simulink model "pidcontrollers"  (R2023a)
settings: Solver=FixedStepAuto  StartTime=0.0  StopTime=50  RelTol=1e-3  EnableMultiTasking=on
settings Model: Creator=dell  LastModifiedBy=mluser
settings SolverCC: AlgebraicLoopSolver=TrustRegion
settings DataIOCC: LimitDataPoints=on  SaveFormat=Array  ReturnWorkspaceOutputs=off
settings OptimizationCC: LifeSpan=inf
settings DebuggingCC: SignalInfNanChecking=error  UnconnectedInputMsg=warning  UnconnectedOutputMsg=warning  UnconnectedLineMsg=warning  SFUnexpectedBacktrackingDiag=warning  SFNoUnconditionalDefaultTransitionDiag=warning  SFExecutionAtInitializationDiag=none  ArithmeticOperatorsInVariantConditions=warning
settings HardwareCC: ProdBitPerPointer=32  ProdBitPerSizeT=32  ProdBitPerPtrDiffT=32  ProdLargestAtomicFloat=None  ProdIntDivRoundTo=Undefined  ProdEndianess=Unspecified  ProdWordSize=32  ProdHWDeviceType=32-bit Generic
settings ModelReferenceCC: PropagateSignalLabelsOutOfModel=off
settings SFSimCC: SimUseLocalCustomCode=off  CustomCodeUndefinedFunction=UseInterfaceOnly
settings RTWCC: RTWUseLocalCustomCode=off
settings CodeAppCC: StateflowObjectComments=on
settings GRTTargetCC: TargetLangStandard=C89/C90 (ANSI)
settings ConfigComp: CovMetricSettings=dw  CovSaveCumulativeToWorkspaceVar=on  CovSaveSingleToWorkspaceVar=on  CovExternalEMLEnable=off

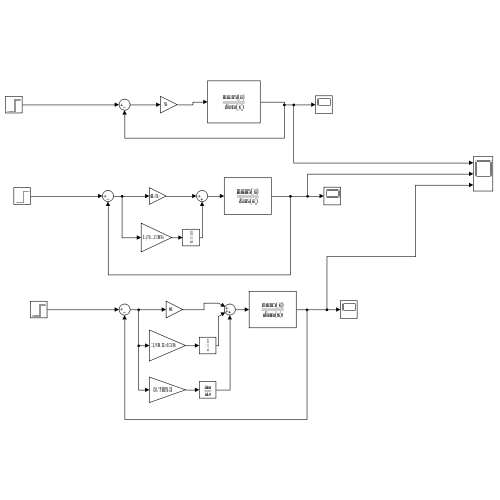
[thumbnail: Simulink's stored preview of the top-level diagram]
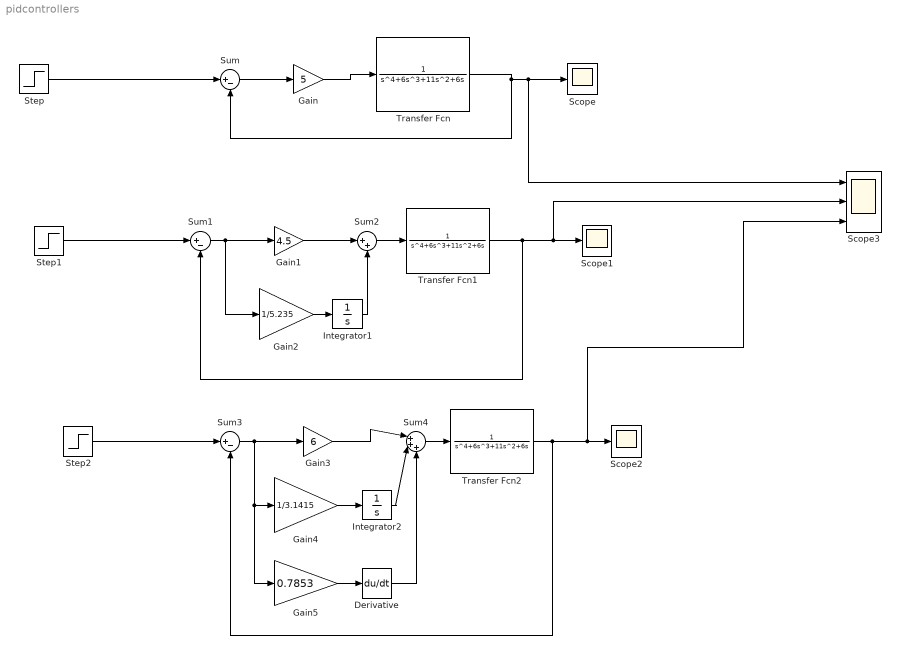
== system pidcontrollers ==
  Derivative : Derivative
  Gain : Gain  Gain=5
  Gain1 : Gain  Gain=4.5
  Gain2 : Gain  Gain=1/5.235
  Gain3 : Gain  Gain=6
  Gain4 : Gain  Gain=1/3.1415
  Gain5 : Gain  Gain=0.7853
  Integrator1 : Integrator
  Integrator2 : Integrator
  Scope : Scope
  Scope1 : Scope
  Scope2 : Scope
  Scope3 : Scope  NumInputPorts=3
  Step : Step  SampleTime=0
  Step1 : Step  SampleTime=0
  Step2 : Step  SampleTime=0
  Sum : Sum  Inputs=|+-
  Sum1 : Sum  Inputs=|+-
  Sum2 : Sum  Inputs=|++
  Sum3 : Sum  Inputs=|+-
  Sum4 : Sum  Inputs=|+++
  Transfer Fcn : TransferFcn  Denominator=[1 6 11 6 0]
  Transfer Fcn1 : TransferFcn  Denominator=[1 6 11 6 0]
  Transfer Fcn2 : TransferFcn  Denominator=[1 6 11 6 0]
  wires:
  Step/1 -> Sum/1
  Sum/1 -> Gain/1
  Gain/1 -> Transfer Fcn/1
  Transfer Fcn/1 -> Sum/2, Scope3/1, Scope/1
  Step1/1 -> Sum1/1
  Sum1/1 -> Gain2/1, Gain1/1
  Gain2/1 -> Integrator1/1
  Integrator1/1 -> Sum2/2
  Gain1/1 -> Sum2/1
  Sum2/1 -> Transfer Fcn1/1
  Transfer Fcn1/1 -> Sum1/2, Scope3/2, Scope1/1
  Step2/1 -> Sum3/1
  Sum3/1 -> Gain5/1, Gain4/1, Gain3/1
  Gain4/1 -> Integrator2/1
  Transfer Fcn2/1 -> Sum3/2, Scope3/3, Scope2/1
  Gain5/1 -> Derivative/1
  Sum4/1 -> Transfer Fcn2/1
  Gain3/1 -> Sum4/1
  Integrator2/1 -> Sum4/2
  Derivative/1 -> Sum4/3
